simulink model "lab1v1.1Orozco"  (R2017b)
settings: Solver=VariableStepAuto  StartTime=0.0  StopTime=3  RelTol=1e-3
undefined symbols (not defined in the file or in its folder): DiscIntNeverNeededParam, magnitude
libraries: simulink_extras x7, commutil2 x5, commchan3 x4, commrandsrc3 x4, simulink x4
settings Model: Creator=n0b0dy  LastModifiedBy=user

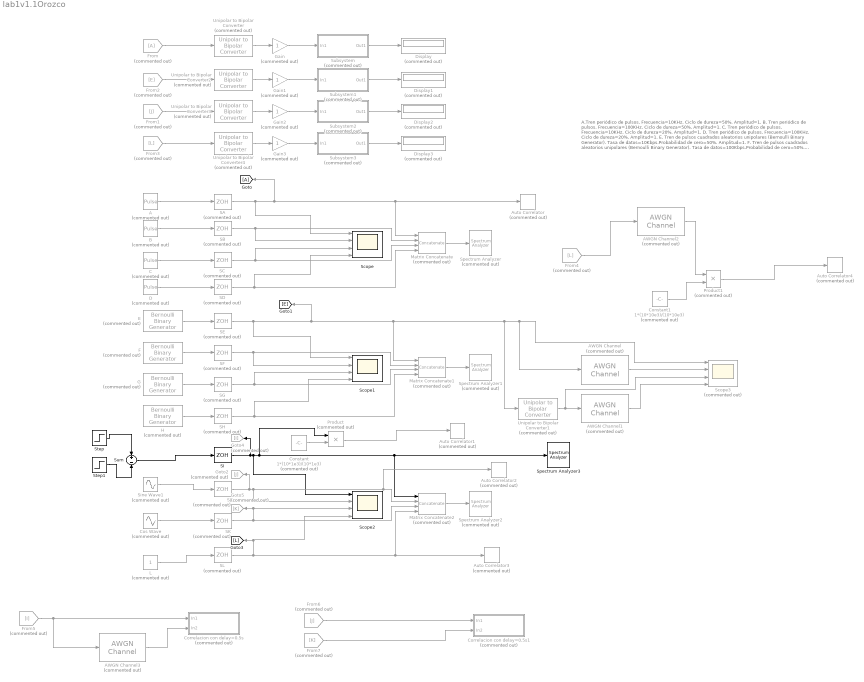
== system lab1v1.1Orozco ==
  note: A.Tren periódico de pulsos. Frecuencia=10KHz. Ciclo de dureza=50%. Amplitud=1.
      | B. Tren periódico de pulsos. Frecuencia=100KHz. Ciclo de dureza=50%. Amplitud=1.
      | C. Tren periódico de pulsos. Frecuencia=10KHz. Ciclo de dureza=20%. Amplitud=1.
      | D. Tren periódico de pulsos. Frecuencia=100KHz. Ciclo de dureza=20%. Amplitud=1.
      | E. Tren de pulsos cuadrados aleatorios unipolares (Bernoulli Binary Generator). Tasa de datos=10Kbps.Probabilidad de cero=50%. Amplitud=1.
      | F. Tren de pulsos cuadrados aleatorios unipolares (Bernoulli Binary Generator). Tasa de datos=100Kbps.Probabilidad de cero=50%. Amplitud=1.
      | G. Tren de pulsos cuadrados aleatorios unipolares (Bernoulli Binary Generator). Tasa de datos=10Kbps.Probabilidad de cero=30%. Amplitud=1.
      | H. Tren de pulsos cuadrados aleatorios unipolares (Bernoulli Binary Generator). Tasa de datos=100Kbps.Probabilidad de cero=30%. Amplitud=1.
      | I. Un pulso rectangular de amplitud 3, iniciando en t0=0.5s y terminando en t1=0.7s
      | J. Seno. Frecuencia=1Khz. Amplitud=1.
      | K. Coseno. Frecuencia=1Khz. Amplitud=1.
      | L. Señal constante. Amplitud=1
  A : DiscretePulseGenerator  Commented=on  PulseType=Time based  Period=1/10E3  PulseWidth=50
  AWGN Channel : commchan3/AWGN Channel  Commented=on  InputProcessing=Columns as channels (frame based)  seed=67  noiseMode="Signal to noise ratio  (SNR)"  EbNodB=10  EsNodB=10  SNRdB=10  bitsPerSym=1  Ps=1  Tsym=1  variance=1
  AWGN Channel1 : commchan3/AWGN Channel  Commented=on  InputProcessing=Columns as channels (frame based)  seed=67  noiseMode="Signal to noise ratio  (SNR)"  EbNodB=10  EsNodB=10  SNRdB=10  bitsPerSym=1  Ps=1  Tsym=1  variance=1
  AWGN Channel2 : commchan3/AWGN Channel  Commented=on  InputProcessing=Columns as channels (frame based)  seed=67  noiseMode="Signal to noise ratio  (SNR)"  EbNodB=10  EsNodB=10  SNRdB=10  bitsPerSym=1  Ps=1  Tsym=1  variance=1
  AWGN Channel3 : commchan3/AWGN Channel  Commented=on  InputProcessing=Columns as channels (frame based)  seed=67  noiseMode="Signal to noise ratio  (SNR)"  EbNodB=10  EsNodB=10  SNRdB=5  bitsPerSym=1  Ps=1  Tsym=1  variance=1
  Auto Correlator : simulink_extras/Additional Sinks/Auto Correlator  Commented=on  npts=1000  HowOften=50  sampleT=1/(10*100e3)
      settings: SourceProductName=Simulink  SourceProductBaseCode=SL
  Auto Correlator1 : simulink_extras/Additional Sinks/Auto Correlator  Commented=on  npts=10000  HowOften=100  sampleT=1/(10*1e3)
      settings: SourceProductName=Simulink  SourceProductBaseCode=SL
  Auto Correlator2 : simulink_extras/Additional Sinks/Auto Correlator  Commented=on  npts=1000  HowOften=50  sampleT=1/(10*100e3)
      settings: SourceProductName=Simulink  SourceProductBaseCode=SL
  Auto Correlator3 : simulink_extras/Additional Sinks/Auto Correlator  Commented=on  npts=1000  HowOften=50  sampleT=1/(10*100e3)
      settings: SourceProductName=Simulink  SourceProductBaseCode=SL
  Auto Correlator4 : simulink_extras/Additional Sinks/Auto Correlator  Commented=on  npts=0.01*(1*100e3)  HowOften=50  sampleT=1/(1*1*100e3)
      settings: SourceProductName=Simulink  SourceProductBaseCode=SL
  B : DiscretePulseGenerator  Commented=on  PulseType=Time based  Period=1/100E3  PulseWidth=50  VectorParams1D=off
  C : DiscretePulseGenerator  Commented=on  PulseType=Time based  Period=1/10E3  PulseWidth=20
  Constant : Constant  Commented=on  Value=1*(10*1e3)/(10*1e3)
  Constant1 : Constant  Commented=on  Value=1*(10*10e3)/(10*10e3)  VectorParams1D=off
  Correlacion con delay=0.5s : Subsystem  Commented=on
  Correlacion con delay=0.5s1 : Subsystem  Commented=on
  Cos Wave : Sin  Commented=on  Frequency=1e3*2*pi  Phase=pi/2  SampleTime=0
      settings: AttributesFormatString=|
      | Frecuency = %<Frequency>
      | Phase = %<Phase>
  D : DiscretePulseGenerator  Commented=on  PulseType=Time based  Period=1/100E3  PulseWidth=20
  Display{,1..3} (4 alike) : Display  Commented=on
  E : commrandsrc3/Bernoulli Binary Generator  Commented=on  ProbabilityOfZero=0.5  SeedSource=Parameter  Seed=1  SampleTime=1/10e3  SamplesPerFrame=1  OutputDataType=double  SimulateUsing=Interpreted execution
  F : commrandsrc3/Bernoulli Binary Generator  Commented=on  ProbabilityOfZero=0.5  SeedSource=Parameter  Seed=1  SampleTime=1/100e3  SamplesPerFrame=1  OutputDataType=double  SimulateUsing=Interpreted execution
  From : From  Commented=on
  From1 : From  Commented=on  GotoTag=J
  From2 : From  Commented=on  GotoTag=E
  From3 : From  Commented=on  GotoTag=L
  From4 : From  Commented=on  GotoTag=L
  From5 : From  Commented=on  GotoTag=I
  From6 : From  Commented=on  GotoTag=J
  From7 : From  Commented=on  GotoTag=K
  G : commrandsrc3/Bernoulli Binary Generator  Commented=on  ProbabilityOfZero=0.3  SeedSource=Parameter  Seed=1  SampleTime=1/10e3  SamplesPerFrame=1  OutputDataType=double  SimulateUsing=Interpreted execution
  Gain{,1..3} (4 alike) : Gain  Commented=on
  Goto2 : Goto  Commented=on  GotoTag=J
  Goto4 : Goto  Commented=on  GotoTag=I
  Goto5 : Goto  Commented=on  GotoTag=K
  H : commrandsrc3/Bernoulli Binary Generator  Commented=on  ProbabilityOfZero=0.3  SeedSource=Parameter  Seed=1  SampleTime=1/100e3  SamplesPerFrame=1  OutputDataType=double  SimulateUsing=Interpreted execution
  L : Constant  Commented=on  SampleTime=1/(6*(1000*2*pi))
  Matrix Concatenate : Concatenate  Commented=on  NumInputs=4  Mode=Multidimensional array  ConcatenateDimension=2
  Matrix Concatenate1 : Concatenate  Commented=on  NumInputs=4  Mode=Multidimensional array  ConcatenateDimension=2
  Matrix Concatenate2 : Concatenate  Commented=on  NumInputs=4  Mode=Multidimensional array  ConcatenateDimension=2
  Product : Product  Commented=on
  Product1 : Product  Commented=on
  SA : ZeroOrderHold  Commented=on  SampleTime=1/(10*100e3)
  SB : ZeroOrderHold  Commented=on  SampleTime=1/(10*100e3)
  SC : ZeroOrderHold  Commented=on  SampleTime=1/(10*100e3)
  SD : ZeroOrderHold  Commented=on  SampleTime=1/(10*100e3)
  SE : ZeroOrderHold  Commented=on  SampleTime=1/(10*10e3)
  SF : ZeroOrderHold  Commented=on  SampleTime=1/(10*100e3)
  SG : ZeroOrderHold  Commented=on  SampleTime=1/(10*100e3)
  SH : ZeroOrderHold  Commented=on  SampleTime=1/(10*100e3)
  SI : ZeroOrderHold  SampleTime=1/(1*1e3)
  SJ : ZeroOrderHold  Commented=on  SampleTime=1/(1*100e3)
  SK : ZeroOrderHold  Commented=on  SampleTime=1/(10*100e3)
  SL : ZeroOrderHold  Commented=on  SampleTime=1/(1*100e3)
  Scope : Scope  NumInputPorts=4
  Scope1 : Scope  NumInputPorts=4
  Scope2 : Scope  NumInputPorts=4
  Scope3 : Scope  Commented=on  NumInputPorts=4
  Sine Wave1 : Sin  Commented=on  Frequency=1e3*2*pi  SampleTime=0
      settings: AttributesFormatString=|
      | Frecuency = %<Frequency>
      | Phase = %<Phase>
  Spectrum Analyzer : SpectrumAnalyzer  Commented=on
  Spectrum Analyzer1 : SpectrumAnalyzer  Commented=on
  Spectrum Analyzer2 : SpectrumAnalyzer  Commented=on
  Spectrum Analyzer3 : SpectrumAnalyzer
  Step : Step  Time=0.5  After=3  SampleTime=1e-3
      settings: AttributesFormatString=Step Time = %<Time>
  Step1 : Step  Time=0.7  After=3  SampleTime=1e-3
      settings: AttributesFormatString=Step Time = %<Time>
  Subsystem : Subsystem  Commented=on
  Subsystem1 : Subsystem  Commented=on
  Subsystem2 : Subsystem  Commented=on
  Subsystem3 : Subsystem  Commented=on
  Sum : Sum  Inputs=+|-
  Unipolar to Bipolar Converter{,2..4} (4 alike) : commutil2/Unipolar to Bipolar Converter  Commented=on  M=4  polarity=Positive  dataType=Inherit via internal rule
      settings: SourceProductName=Communications System Toolbox
  Unipolar to Bipolar Converter1 : commutil2/Unipolar to Bipolar Converter  Commented=on  M=2  polarity=Positive  dataType=Inherit via internal rule
      settings: SourceProductName=Communications System Toolbox
  wires:
  A/1 -> SA/1
  E/1 -> SE/1
  F/1 -> SF/1
  G/1 -> SG/1
  H/1 -> SH/1
  B/1 -> SB/1
  C/1 -> SC/1
  D/1 -> SD/1
  SA/1 -> Scope/1, [A], Auto Correlator/1, Matrix Concatenate/1
  SD/1 -> Matrix Concatenate/4, Scope/4
  SH/1 -> Matrix Concatenate1/4, Scope1/4
  SG/1 -> Matrix Concatenate1/3, Scope1/3
  SF/1 -> Matrix Concatenate1/2, Scope1/2
  Matrix Concatenate1/1 -> Spectrum Analyzer1/1
  SC/1 -> Scope/3, Matrix Concatenate/3
  SB/1 -> Scope/2, Matrix Concatenate/2
  L/1 -> SL/1
  Sine Wave1/1 -> SJ/1
  Cos Wave/1 -> SK/1
  SI/1 -> Goto4/1, Scope2/1, Product/1, Spectrum Analyzer3/1, Matrix Concatenate2/1
  SJ/1 -> Goto2/1, Scope2/2, Auto Correlator2/1, Matrix Concatenate2/2
  SK/1 -> Goto5/1, Scope2/3, Matrix Concatenate2/3
  SL/1 -> [L], Scope2/4, Auto Correlator3/1, Matrix Concatenate2/4
  Matrix Concatenate2/1 -> Spectrum Analyzer2/1
  Matrix Concatenate/1 -> Spectrum Analyzer/1
  Unipolar to Bipolar Converter/1 -> Gain/1
  Gain/1 -> Subsystem/1(In1)
  Subsystem/1(Out1) -> Display/1
  AWGN Channel/1 -> Scope3/2
  Unipolar to Bipolar Converter1/1 -> Scope3/3, AWGN Channel1/1
  AWGN Channel1/1 -> Scope3/4
  From/1 -> Unipolar to Bipolar Converter/1
  Subsystem1/1(Out1) -> Display1/1
  Gain1/1 -> Subsystem1/1(In1)
  Unipolar to Bipolar Converter2/1 -> Gain1/1
  From2/1 -> Unipolar to Bipolar Converter2/1
  Subsystem2/1(Out1) -> Display2/1
  Gain2/1 -> Subsystem2/1(In1)
  Unipolar to Bipolar Converter3/1 -> Gain2/1
  From1/1 -> Unipolar to Bipolar Converter3/1
  Subsystem3/1(Out1) -> Display3/1
  Gain3/1 -> Subsystem3/1(In1)
  Unipolar to Bipolar Converter4/1 -> Gain3/1
  From3/1 -> Unipolar to Bipolar Converter4/1
  Step1/1 -> Sum/2
  Step/1 -> Sum/1
  Sum/1 -> SI/1
  Constant/1 -> Product/2
  Product/1 -> Auto Correlator1/1
  Constant1/1 -> Product1/2
  Product1/1 -> Auto Correlator4/1
  SE/1 -> [E], Matrix Concatenate1/1, Unipolar to Bipolar Converter1/1, AWGN Channel/1, Scope3/1, Scope1/1
  From4/1 -> AWGN Channel2/1
  AWGN Channel2/1 -> Product1/1
  From5/1 -> AWGN Channel3/1, Correlacion con delay=0.5s/1(In1)
  AWGN Channel3/1 -> Correlacion con delay=0.5s/2(In2)
  From6/1 -> Correlacion con delay=0.5s1/1(In1)
  From7/1 -> Correlacion con delay=0.5s1/2(In2)

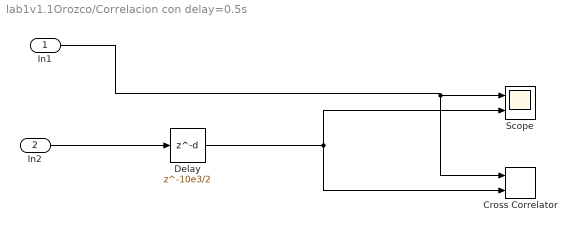
== system lab1v1.1Orozco/Correlacion con delay=0.5s ==
  In1 : Inport
  In2 : Inport  Port=2
  Cross Correlator : simulink_extras/Additional Sinks/Cross Correlator  npts=2*(10*1e3)  HowOften=50  sampleT=1/(10*1e3)
      settings: SourceProductName=Simulink  SourceProductBaseCode=SL
  Delay : Delay  DelayLength=10e3/2  InitialCondition=0
  Scope : Scope  NumInputPorts=2
  wires:
  In1/1 -> Cross Correlator/1, Scope/1
  Delay/1 -> Cross Correlator/2, Scope/2
  In2/1 -> Delay/1

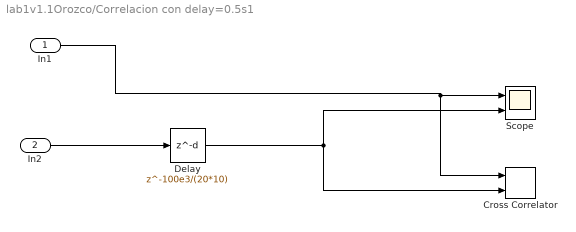
== system lab1v1.1Orozco/Correlacion con delay=0.5s1 ==
  In1 : Inport
  In2 : Inport  Port=2
  Cross Correlator : simulink_extras/Additional Sinks/Cross Correlator  npts=0.01*(1*100e3)  HowOften=50  sampleT=1/(100*1e3)
      settings: SourceProductName=Simulink  SourceProductBaseCode=SL
  Delay : Delay  DelayLength=100e3/(20*10)  InitialCondition=0
  Scope : Scope  NumInputPorts=2
  wires:
  In1/1 -> Cross Correlator/1, Scope/1
  Delay/1 -> Cross Correlator/2, Scope/2
  In2/1 -> Delay/1

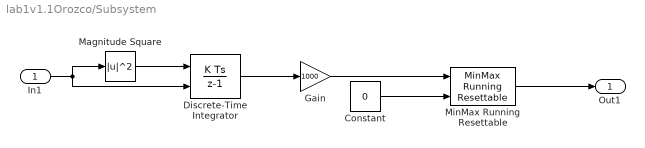
== system lab1v1.1Orozco/Subsystem ==
  In1 : Inport
  Constant : Constant  Value=0
  Discrete-Time Integrator : DiscreteIntegrator  gainval=1000  ExternalReset=rising  InitialConditionSetting=State (most efficient)  SampleTime=-1  ICPrevOutput=DiscIntNeverNeededParam  ICPrevScaledInput=DiscIntNeverNeededParam
  Gain : Gain  Gain=1000
  Magnitude Square : Math  Operator=magnitude^2  RndMeth=Zero  SaturateOnIntegerOverflow=on
  MinMax Running Resettable : simulink/Math Operations/MinMax Running Resettable  Function=min  vinit=0.0
  Out1 : Outport
  wires:
  In1/1 -> Discrete-Time Integrator/2, Magnitude Square/1
  MinMax Running Resettable/1 -> Out1/1
  Gain/1 -> MinMax Running Resettable/1
  Constant/1 -> MinMax Running Resettable/2
  Magnitude Square/1 -> Discrete-Time Integrator/1
  Discrete-Time Integrator/1 -> Gain/1

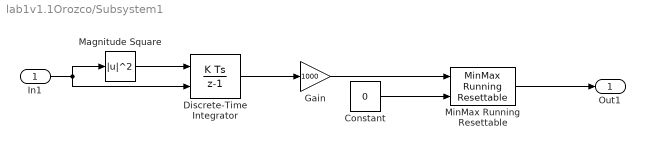
== system lab1v1.1Orozco/Subsystem1 ==
  In1 : Inport
  Constant : Constant  Value=0
  Discrete-Time Integrator : DiscreteIntegrator  gainval=1000  ExternalReset=rising  InitialConditionSetting=State (most efficient)  SampleTime=-1  ICPrevOutput=DiscIntNeverNeededParam  ICPrevScaledInput=DiscIntNeverNeededParam
  Gain : Gain  Gain=1000
  Magnitude Square : Math  Operator=magnitude^2  RndMeth=Zero  SaturateOnIntegerOverflow=on
  MinMax Running Resettable : simulink/Math Operations/MinMax Running Resettable  Function=min  vinit=0.0
  Out1 : Outport
  wires:
  In1/1 -> Discrete-Time Integrator/2, Magnitude Square/1
  MinMax Running Resettable/1 -> Out1/1
  Gain/1 -> MinMax Running Resettable/1
  Constant/1 -> MinMax Running Resettable/2
  Magnitude Square/1 -> Discrete-Time Integrator/1
  Discrete-Time Integrator/1 -> Gain/1

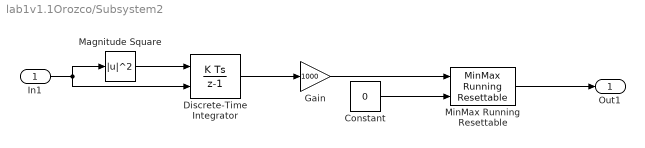
== system lab1v1.1Orozco/Subsystem2 ==
  In1 : Inport
  Constant : Constant  Value=0
  Discrete-Time Integrator : DiscreteIntegrator  gainval=1000  ExternalReset=rising  InitialConditionSetting=State (most efficient)  SampleTime=-1  ICPrevOutput=DiscIntNeverNeededParam  ICPrevScaledInput=DiscIntNeverNeededParam
  Gain : Gain  Gain=1000
  Magnitude Square : Math  Operator=magnitude^2  RndMeth=Zero  SaturateOnIntegerOverflow=on
  MinMax Running Resettable : simulink/Math Operations/MinMax Running Resettable  Function=min  vinit=0.0
  Out1 : Outport
  wires:
  In1/1 -> Discrete-Time Integrator/2, Magnitude Square/1
  MinMax Running Resettable/1 -> Out1/1
  Gain/1 -> MinMax Running Resettable/1
  Constant/1 -> MinMax Running Resettable/2
  Magnitude Square/1 -> Discrete-Time Integrator/1
  Discrete-Time Integrator/1 -> Gain/1

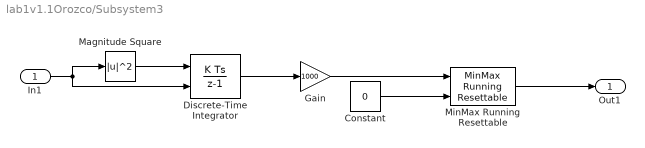
== system lab1v1.1Orozco/Subsystem3 ==
  In1 : Inport
  Constant : Constant  Value=0
  Discrete-Time Integrator : DiscreteIntegrator  gainval=1000  ExternalReset=rising  InitialConditionSetting=State (most efficient)  SampleTime=-1  ICPrevOutput=DiscIntNeverNeededParam  ICPrevScaledInput=DiscIntNeverNeededParam
  Gain : Gain  Gain=1000
  Magnitude Square : Math  Operator=magnitude^2  RndMeth=Zero  SaturateOnIntegerOverflow=on
  MinMax Running Resettable : simulink/Math Operations/MinMax Running Resettable  Function=min  vinit=0.0
  Out1 : Outport
  wires:
  In1/1 -> Discrete-Time Integrator/2, Magnitude Square/1
  MinMax Running Resettable/1 -> Out1/1
  Gain/1 -> MinMax Running Resettable/1
  Constant/1 -> MinMax Running Resettable/2
  Magnitude Square/1 -> Discrete-Time Integrator/1
  Discrete-Time Integrator/1 -> Gain/1
